simulink model "rockymodel"  (R2020b)
settings: Solver=VariableStepAuto  StartTime=0.0  StopTime=30  RelTol=1e-3
values from neighbouring files (symbols this model uses):
  g = 9.81    [Rocky_closed_loop_poles.m]    (also in control_parameters.m)
  Ki = double(solutions.Ki)    [Rocky_closed_loop_poles.m]    (also in control_parameters.m = real(double(solutions.Ki)))
  Kp = double(solutions.Kp)    [Rocky_closed_loop_poles.m]    (also in control_parameters.m = real(double(solutions.Kp)))
  l_eff = 9.81/(wn^2)    [gyroscope_parameters.m]
  tau = coeffs.b1    [motor_parameters.m]
undefined symbols (not defined in the file or in its folder): K_motor
libraries: simulink x1
settings Model: Creator=nolan  LastModifiedBy=nolan

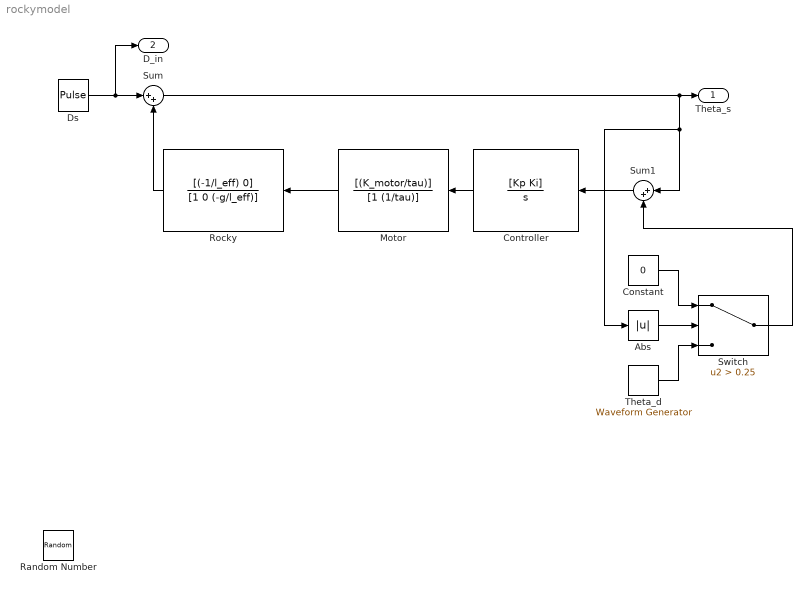
== system rockymodel ==
  Abs : Abs
  Constant : Constant  Value=0
  Controller : TransferFcn  Numerator=[Kp Ki]  Denominator=[1 0]
  Ds : DiscretePulseGenerator  PulseType=Time based  Amplitude=0.5  Period=10  PhaseDelay=1
  Motor : TransferFcn  Numerator=[(K_motor/tau)]  Denominator=[1 (1/tau)]
  Random Number : RandomNumber  Variance=0.00000001  SampleTime=0.01
  Rocky : TransferFcn  Numerator=[(-1/l_eff) 0]  Denominator=[1 0 (-g/l_eff)]
  Sum : Sum  Inputs=|++
  Sum1 : Sum  Inputs=|++
  Switch : Switch  Criteria=u2 > Threshold  Threshold=0.25  ZeroCross=off
  Theta_d : simulink/Sources/Waveform Generator  OutMin=[]  OutMax=[]  OutDataTypeStr=double  SelectedSignal=1  Signals=sin(sin(0.1, 1, 0), 20, 0)  BlockNames=MultiportSwitch_79505fb0ea284da  SampleTime=0.1
  Theta_s : Outport
  D_in : Outport  Port=2
  wires:
  Rocky/1 -> Sum/2
  Controller/1 -> Motor/1
  Ds/1 -> D_in/1, Sum/1
  Abs/1 -> Switch/2
  Theta_d/1 -> Switch/3
  Motor/1 -> Rocky/1
  Sum/1 -> Abs/1, Sum1/1, Theta_s/1
  Constant/1 -> Switch/1
  Sum1/1 -> Controller/1
  Switch/1 -> Sum1/2
